simulink model "MotorCtrl_FOC_Math"  (R2025b)
settings: Solver=FixedStepDiscrete  StartTime=0.0  StopTime=5  FixedStep=MC_Sim_BaseStep  RelTol=1e-3  EnableMultiTasking=on
values from neighbouring files (symbols this model uses):
  MC_ADC_BitNum = 0.0    [MotorControlDataDictionary_Math.sldd]
  MC_ADC_Offset = 0.0    [MotorControlDataDictionary_Math.sldd]
  MC_ADC_VRef = 1.0    [MotorControlDataDictionary_Math.sldd]
  MC_CSA_Gain = 1.0    [MotorControlDataDictionary_Math.sldd]
  MC_MOS_DeadTime = 1.3E-6    [MotorControlDataDictionary_Math.sldd]
  MC_Motor_Mechinal_Damp = 1.0E-5    [MotorControlDataDictionary_Math.sldd]
  MC_Motor_Mechinal_Fric = 0.0    [MotorControlDataDictionary_Math.sldd]
  MC_Motor_Mechinal_Inertia = 0.0103    [MotorControlDataDictionary_Math.sldd]
  MC_Motor_Phi = 0.0059190254913385806    [MotorControlDataDictionary_Math.sldd]
  MC_Motor_Rotor_Pn = 4.0    [MotorControlDataDictionary_Math.sldd]
  MC_Motor_Stator_Ld = 5.6345E-5    [MotorControlDataDictionary_Math.sldd]
  MC_Motor_Stator_Lq = 5.6345E-5    [MotorControlDataDictionary_Math.sldd]
  MC_Motor_Stator_Rs = 0.0286    [MotorControlDataDictionary_Math.sldd]
  MC_Param_CurrentPI_Ki = 0.0089705790612839825    [MotorControlDataDictionary_Math.sldd]
  MC_Param_CurrentPI_Kp = 0.283220860906427    [MotorControlDataDictionary_Math.sldd]
  MC_Param_CurrentPI_UdInteMax = 7.794228634059948    [MotorControlDataDictionary_Math.sldd]
  MC_Param_CurrentPI_UdInteMin = -7.794228634059948    [MotorControlDataDictionary_Math.sldd]
  MC_Param_CurrentPI_UdMax = 7.794228634059948    [MotorControlDataDictionary_Math.sldd]
  MC_Param_CurrentPI_UdMin = -7.794228634059948    [MotorControlDataDictionary_Math.sldd]
  MC_Param_CurrentPI_UqInteMax = 7.794228634059948    [MotorControlDataDictionary_Math.sldd]
  MC_Param_CurrentPI_UqInteMin = -7.794228634059948    [MotorControlDataDictionary_Math.sldd]
  MC_Param_CurrentPI_UqMax = 7.794228634059948    [MotorControlDataDictionary_Math.sldd]
  MC_Param_CurrentPI_UqMin = -7.794228634059948    [MotorControlDataDictionary_Math.sldd]
  MC_Param_Flux_Gamma = 750000.0    [MotorControlDataDictionary_Math.sldd]
  MC_Param_Flux_Lalpha = 5.6345E-5    [MotorControlDataDictionary_Math.sldd]
  MC_Param_Flux_Lbeta = 5.6345E-5    [MotorControlDataDictionary_Math.sldd]
  MC_Param_Flux_Ralpha = 0.0286    [MotorControlDataDictionary_Math.sldd]
  MC_Param_Flux_Rbeta = 0.0286    [MotorControlDataDictionary_Math.sldd]
  MC_Param_Luen_BEMFalpha = -17747.803709290976    [MotorControlDataDictionary_Math.sldd]
  MC_Param_Luen_BEMFbeta = -17747.803709290976    [MotorControlDataDictionary_Math.sldd]
  MC_Param_Luen_BEMFErr = 10.0    [MotorControlDataDictionary_Math.sldd]
  MC_Param_Luen_Currentalpha = -507.58718608572195    [MotorControlDataDictionary_Math.sldd]
  MC_Param_Luen_Currentbeta = -507.58718608572195    [MotorControlDataDictionary_Math.sldd]
  MC_Param_Luen_CurrentErr = 400.0    [MotorControlDataDictionary_Math.sldd]
  MC_Param_Luen_PLL_Ki = 0.24634532585119037    [MotorControlDataDictionary_Math.sldd]
  MC_Param_Luen_PLL_Kp = 125.66370614359172    [MotorControlDataDictionary_Math.sldd]
  MC_Param_Luen_Voltagealpha = 17747.803709290976    [MotorControlDataDictionary_Math.sldd]
  MC_Param_Luen_Voltagebeta = 17747.803709290976    [MotorControlDataDictionary_Math.sldd]
  MC_Param_PhasetoReal = 500.0    [MotorControlDataDictionary_Math.sldd]
  MC_Param_SMO_CoffA = 0.968326559588251    [MotorControlDataDictionary_Math.sldd]
  MC_Param_SMO_CoffB = 1.1074629514597569    [MotorControlDataDictionary_Math.sldd]
  MC_Param_SpeedCtrl_IdMax = 60.0    [MotorControlDataDictionary_Math.sldd]
  MC_Param_SpeedCtrl_IdMin = -60.0    [MotorControlDataDictionary_Math.sldd]
  MC_Param_SpeedCtrl_IqMax = 60.0    [MotorControlDataDictionary_Math.sldd]
  MC_Param_SpeedCtrl_IqMin = -60.0    [MotorControlDataDictionary_Math.sldd]
  MC_Param_SpeedPI_Ki = 0.57157085739428382    [MotorControlDataDictionary_Math.sldd]
  MC_Param_SpeedPI_Kp = 9.1114109857344836    [MotorControlDataDictionary_Math.sldd]
  MC_Param_SpeedtoTheta = 6.24E-5    [MotorControlDataDictionary_Math.sldd]
  MC_Param_SVPWM_DutyMax = 0.98    [MotorControlDataDictionary_Math.sldd]
  MC_Param_SVPWM_DutyMin = 0.02    [MotorControlDataDictionary_Math.sldd]
  MC_Param_SVPWM_SampleOffset1 = 0.02    [MotorControlDataDictionary_Math.sldd]
  MC_Param_SVPWM_SampleOffset2 = 0.015    [MotorControlDataDictionary_Math.sldd]
  MC_Param_SVPWM_SampleValid = 0.0096153846153846159    [MotorControlDataDictionary_Math.sldd]
  MC_Param_Zero = 0.0    [MotorControlDataDictionary_Math.sldd]
  MC_Sample_CurrentNoise = 1.0E-15    [MotorControlDataDictionary_Math.sldd]
  MC_Sample_Rs = 0.002    [MotorControlDataDictionary_Math.sldd]
  MC_Sample_VbusNoise = 1.0E-15    [MotorControlDataDictionary_Math.sldd]
  MC_Sim_BaseStep = 2.08E-8    [MotorControlDataDictionary_Math.sldd]
  MC_Sim_HFTStep = 6.24E-5    [MotorControlDataDictionary_Math.sldd]
  MC_Sim_MFTStep = 0.0019968    [MotorControlDataDictionary_Math.sldd]
libraries: simulink x28, nesl_utility x19, fl_lib x14, ee_lib x13, autolibpmsminterior x2, autolibinverter x1
(part 2 of 8)

== system MotorCtrl_FOC_Math/Tracking-Differentiator ==
  Ref_In : Inport
  Add : Sum
  Add1 : Sum
  Delay One Step : Delay  DelayLength=1  InitialCondition=MC_Param_Zero
  Delay One Step1 : Delay  DelayLength=1  InitialCondition=MC_Param_Zero
  Gain : Gain  Gain=MC_Sim_MFTStep  ParamDataTypeStr=single  OutDataTypeStr=single  RndMeth=Simplest
  Gain1 : Gain  Gain=MC_Sim_MFTStep  OutDataTypeStr=single  RndMeth=Simplest
  Signal Copy : SignalConversion  OverrideOpt=off
  fastFunc1_TD : Subsystem  Commented=on
  fastFunc2_TD : Subsystem
  SpeedTarget_TD : Outport
  wires:
  Ref_In/1 -> fastFunc2_TD/1(Ref_In), fastFunc1_TD/1(Ref_In)
  fastFunc2_TD/1(Ref_TD) -> Gain/1  "u"
  Add/1 -> Gain1/1, Delay One Step/1  "x2"
  Delay One Step/1 -> Add/2, [x2_delay]
  Gain/1 -> Add/1  "T*u"
  Gain1/1 -> Add1/1  "T*x2"
  Add1/1 -> Signal Copy/1, Delay One Step1/1  "x1"
  Delay One Step1/1 -> Add1/2, [x1_delay]
  Signal Copy/1 -> SpeedTarget_TD/1  "SpeedTarget_TD"
  [x1_delay] -> fastFunc2_TD/2(X1), fastFunc1_TD/2(X1)
  [x2_delay] -> fastFunc2_TD/3(X2), fastFunc1_TD/3(X2)

== system MotorCtrl_FOC_Math/HFTask/LuenbergerObservor ==
  Valpha : Inport
  Vbeta : Inport  Port=2
  Ialpha : Inport  Port=3
  Ibeta : Inport  Port=4
  We : Inport  Port=5
  Delay One Step : Delay  DelayLength=1  InitialCondition=single(0)
  Terminator : Terminator
  getE : Subsystem
  getSpeedandTheta : Subsystem
  Speed : Outport
  Theta : Outport  Port=2
  wires:
  getSpeedandTheta/2(Theta) -> Theta/1
  getSpeedandTheta/1(Speed) -> Speed/1
  getE/2(Ebeta) -> getSpeedandTheta/2(Ebeta)
  getE/1(Ealpha) -> getSpeedandTheta/1(Ealpha)
  Ibeta/1 -> getE/4(Ibeta)
  Ialpha/1 -> getE/3(Ialpha)
  Vbeta/1 -> getE/2(Vbeta)
  Valpha/1 -> getE/1(Valpha)
  getSpeedandTheta/3(We) -> Delay One Step/1
  We/1 -> Terminator/1
  Delay One Step/1 -> getE/5(We)

== system MotorCtrl_FOC_Math/HFTask/axisTransform ==
  Ia : Inport
  Ib : Inport  Port=2
  SinTheta : Inport  Port=3
  CosTheta : Inport  Port=4
  Add1 : Sum
  Product{,1..3} (4 alike) : Product
  Signal Copy : SignalConversion  OverrideOpt=off
  Subtract : Sum  Inputs=-+
  a_plus_2b : Sum  Inputs=+++  RndMeth=Simplest  OutDataTypeStr=Inherit: Same as first input
  one_by_sqrt3 : Gain  Gain=1/sqrt(3)  RndMeth=Simplest  OutDataTypeStr=Inherit: Same as input
  Ialpha : Outport
  Ibeta : Outport  Port=2
  Id : Outport  Port=3
  Iq : Outport  Port=4
  wires:
  Product3/1 -> Subtract/2
  Product2/1 -> Subtract/1
  Add1/1 -> Id/1  "Id"
  Subtract/1 -> Iq/1  "Iq"
  Product/1 -> Add1/1
  Product1/1 -> Add1/2
  CosTheta/1 -> Product3/2, Product/2
  SinTheta/1 -> Product2/2, Product1/2
  a_plus_2b/1 -> one_by_sqrt3/1
  one_by_sqrt3/1 -> Ibeta/1, Product3/1, Product1/1  "Ibeta"
  Signal Copy/1 -> Ialpha/1, Product2/1, Product/1  "Ialpha"
  Ia/1 -> a_plus_2b/1, Signal Copy/1
  Ib/1 -> a_plus_2b/3, a_plus_2b/2

== system MotorCtrl_FOC_Math/HFTask/currentADRC ==
  note: ADRC开发日志:
      | 20251229：
      | 感觉观测器参数存在问题，观测值瞬间会和参考值相等，导致PI控制器调节电流增速较慢
      | 2026.01.05
      | 1、LESO中的两个fal函数出现周期性震荡
      | 2、NLSEF中的电压输出值只有1.xV，电机转速无法提升
      | 2026.01.07
      | 1、减小NLSEF的参数，可以实现系统的收敛，且效果与PI控制器类似
  IdRef : Inport
  IqRef : Inport  Port=2
  Id : Inport  Port=3
  Iq : Inport  Port=4
  Ud : Inport  Port=5
  Uq : Inport  Port=6
  IntregralResetFlag : Inport  Port=7
  Wm : Inport  Port=8
  Delay One Step : Delay  InitialCondition=single(0)
  Delay One Step1 : Delay  InitialCondition=single(0)
  LESO : Subsystem  VariantControl=ESO
  NLSEF : Subsystem  VariantControl=NLSEF
  Terminator : Terminator
  UdRef : Outport
  UqRef : Outport  Port=2
  wires:
  NLSEF/1(Ud_ADRC) -> UdRef/1  "UdRef"
  NLSEF/2(Uq_ADRC) -> UqRef/1  "UqRef"
  IdRef/1 -> NLSEF/1(Id_Ref)
  Id/1 -> LESO/1(Id)
  IqRef/1 -> NLSEF/2(Iq_Ref)
  Iq/1 -> LESO/3(Iq)
  IntregralResetFlag/1 -> Terminator/1
  Delay One Step/1 -> LESO/2(Ud)
  Delay One Step1/1 -> LESO/4(Uq)
  LESO/2(Iq_ESO) -> NLSEF/4(Iq_ESO)
  LESO/1(Id_ESO) -> NLSEF/3(Id_ESO)
  LESO/3(Id_Dis) -> NLSEF/5(Id_ESO_Dis)
  LESO/4(Iq_Dis) -> NLSEF/6(Iq_ESO_Dis)
  Ud/1 -> Delay One Step/1
  Uq/1 -> Delay One Step1/1

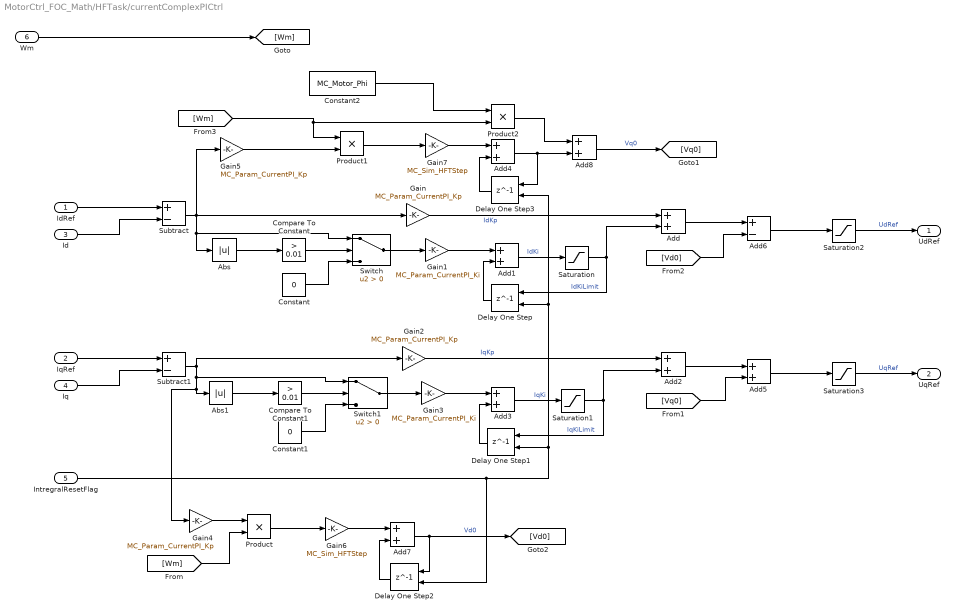
== system MotorCtrl_FOC_Math/HFTask/currentComplexPICtrl ==
  IdRef : Inport
  IqRef : Inport  Port=2
  Id : Inport  Port=3
  Iq : Inport  Port=4
  IntregralResetFlag : Inport  Port=5
  Wm : Inport  Port=6
  Abs : Abs  SaturateOnIntegerOverflow=off
  Abs1 : Abs  SaturateOnIntegerOverflow=off
  Add{,2,5,8} (4 alike) : Sum
  Add{1,3..4,7} (4 alike) : Sum  OutDataTypeStr=single
  Add6 : Sum  Inputs=+-
  Compare To Constant : simulink/Logic and Bit Operations/Compare To Constant  relop=>  const=0.01  OutDataTypeStr=boolean
  Compare To Constant1 : simulink/Logic and Bit Operations/Compare To Constant  relop=>  const=0.01  OutDataTypeStr=boolean
  Constant : Constant  Value=0  OutDataTypeStr=single
  Constant1 : Constant  Value=0  OutDataTypeStr=single
  Constant2 : Constant  Value=MC_Motor_Phi  OutDataTypeStr=single
  Delay One Step{,1..3} (4 alike) : Delay  DelayLength=1  ExternalReset=Level
      settings: InputPortMap=u0,r5
  Gain : Gain  Gain=MC_Param_CurrentPI_Kp  OutDataTypeStr=single
  Gain1 : Gain  Gain=MC_Param_CurrentPI_Ki  OutDataTypeStr=single
  Gain2 : Gain  Gain=MC_Param_CurrentPI_Kp  OutDataTypeStr=single
  Gain3 : Gain  Gain=MC_Param_CurrentPI_Ki  OutDataTypeStr=single
  Gain4 : Gain  Gain=MC_Param_CurrentPI_Kp
  Gain5 : Gain  Gain=MC_Param_CurrentPI_Kp
  Gain6 : Gain  Gain=MC_Sim_HFTStep  OutDataTypeStr=single
  Gain7 : Gain  Gain=MC_Sim_HFTStep  OutDataTypeStr=single
  Product : Product
  Product1 : Product
  Product2 : Product
  Saturation : Saturate  UpperLimit=MC_Param_CurrentPI_UdInteMax  LowerLimit=MC_Param_CurrentPI_UdInteMin
  Saturation1 : Saturate  UpperLimit=MC_Param_CurrentPI_UqInteMax  LowerLimit=MC_Param_CurrentPI_UqInteMin
  Saturation2 : Saturate  UpperLimit=MC_Param_CurrentPI_UdMax  LowerLimit=MC_Param_CurrentPI_UdMin
  Saturation3 : Saturate  UpperLimit=MC_Param_CurrentPI_UqMax  LowerLimit=MC_Param_CurrentPI_UqMin
  Subtract : Sum  Inputs=+-
  Subtract1 : Sum  Inputs=+-
  Switch : Switch  Criteria=u2 > Threshold  SaturateOnIntegerOverflow=off  InputSameDT=off
  Switch1 : Switch  Criteria=u2 > Threshold  SaturateOnIntegerOverflow=off  InputSameDT=off
  UdRef : Outport
  UqRef : Outport  Port=2
  wires:
  Wm/1 -> [Wm]
  Saturation3/1 -> UqRef/1  "UqRef"
  Saturation2/1 -> UdRef/1  "UdRef"
  [Vd0] -> Add6/2
  Add6/1 -> Saturation2/1
  Add/1 -> Add6/1
  [Vq0] -> Add5/2
  Add2/1 -> Add5/1
  [Wm] -> Product/2
  Id/1 -> Subtract/2
  Gain4/1 -> Product/1
  Switch1/1 -> Gain3/1
  Abs1/1 -> Compare To Constant1/1
  Compare To Constant1/1 -> Switch1/2
  Constant1/1 -> Switch1/3
  Constant/1 -> Switch/3
  Compare To Constant/1 -> Switch/2
  Switch/1 -> Gain1/1
  Add5/1 -> Saturation3/1
  IqRef/1 -> Subtract1/1
  Iq/1 -> Subtract1/2
  Subtract1/1 -> Gain2/1, Gain4/1, Abs1/1, Switch1/1
  Gain2/1 -> Add2/1  "IqKp"
  Gain3/1 -> Add3/1
  Delay One Step1/1 -> Add3/2
  Add3/1 -> Saturation1/1  "IqKi"
  Saturation1/1 -> Add2/2, Delay One Step1/1  "IqKiLimit"
  Saturation/1 -> Delay One Step/1, Add/2  "IdKiLimit"
  Add1/1 -> Saturation/1  "IdKi"
  Delay One Step/1 -> Add1/2
  Gain1/1 -> Add1/1
  Abs/1 -> Compare To Constant/1
  Gain/1 -> Add/1  "IdKp"
  Subtract/1 -> Gain5/1, Abs/1, Switch/1, Gain/1
  IdRef/1 -> Subtract/1
  Gain6/1 -> Add7/1
  Product/1 -> Gain6/1
  Delay One Step2/1 -> Add7/2
  Add7/1 -> [Vd0], Delay One Step2/1  "Vd0"
  Add4/1 -> Delay One Step3/1, Add8/2
  Delay One Step3/1 -> Add4/2
  Gain7/1 -> Add4/1
  IntregralResetFlag/1 -> Delay One Step2/2, Delay One Step1/2, Delay One Step3/2, Delay One Step/2
  Product1/1 -> Gain7/1
  Constant2/1 -> Product2/1
  Gain5/1 -> Product1/2
  Add8/1 -> [Vq0]  "Vq0"
  Product2/1 -> Add8/1
  [Wm] -> Product1/1, Product2/2

== system MotorCtrl_FOC_Math/HFTask/currentDBC ==
  note: 无差拍电流控制器（延时1拍）
  IdRef : Inport
  IqRef : Inport  Port=2
  Id : Inport  Port=3
  Iq : Inport  Port=4
  Wm : Inport  Port=5
  Add5 : Sum  Inputs=++-
  Add6 : Sum  Inputs=+++
  Add7 : Sum
  Constant1 : Constant  Value=MC_Motor_Phi  OutDataTypeStr=single
  Gain10 : Gain  Gain=MC_Motor_Stator_Lq
  Gain11 : Gain  Gain=MC_Motor_Stator_Lq/MC_Sim_HFTStep
  Gain12 : Gain  Gain=MC_Motor_Stator_Rs-(MC_Motor_Stator_Lq/MC_Sim_HFTStep)
  Gain13 : Gain  Gain=MC_Motor_Stator_Ld
  Gain8 : Gain  Gain=MC_Motor_Stator_Ld/MC_Sim_HFTStep
  Gain9 : Gain  Gain=MC_Motor_Stator_Rs-(MC_Motor_Stator_Ld/MC_Sim_HFTStep)
  Product2 : Product
  Product3 : Product
  Saturation : Saturate  UpperLimit=MC_Param_CurrentPI_UdMax  LowerLimit=MC_Param_CurrentPI_UdMin
  Saturation1 : Saturate  UpperLimit=MC_Param_CurrentPI_UqMax  LowerLimit=MC_Param_CurrentPI_UqMin
  UdRef : Outport
  UqRef : Outport  Port=2
  wires:
  Wm/1 -> [Wm]
  Iq/1 -> [Iq]
  Id/1 -> [Id]
  IqRef/1 -> [IqRef]
  IdRef/1 -> [IdRef]
  [IdRef] -> Gain8/1
  Gain8/1 -> Add5/1  "IdRef_Vd"
  [Id] -> Gain9/1
  Gain9/1 -> Add5/2  "Id_Vd"
  [Iq] -> Gain10/1
  Gain10/1 -> Product2/2
  [Wm] -> Product2/1
  [IqRef] -> Gain11/1
  Gain11/1 -> Add6/1  "IqRef_Vq"
  Gain12/1 -> Add6/2  "Iq_Vq"
  [Iq] -> Gain12/1
  [Wm] -> Product3/1
  Add7/1 -> Product3/2
  Constant1/1 -> Add7/2
  Gain13/1 -> Add7/1
  [Id] -> Gain13/1
  Saturation/1 -> UdRef/1  "UdRef_DBC"
  Saturation1/1 -> UqRef/1  "UqRef_DBC"
  Add5/1 -> Saturation/1
  Product2/1 -> Add5/3  "Iq_Vd"
  Add6/1 -> Saturation1/1
  Product3/1 -> Add6/3  "Id_Vq"

== system MotorCtrl_FOC_Math/HFTask/currentPIControl ==
  IdRef : Inport
  IqRef : Inport  Port=2
  Id : Inport  Port=3
  Iq : Inport  Port=4
  IntregralResetFlag : Inport  Port=5
  Wm : Inport  Port=6
  Abs : Abs  SaturateOnIntegerOverflow=off
  Abs1 : Abs  SaturateOnIntegerOverflow=off
  Add{,2,4..5} (4 alike) : Sum
  Add1 : Sum  OutDataTypeStr=single
  Add3 : Sum  OutDataTypeStr=single
  Add6 : Sum  Inputs=+-
  Compare To Constant : simulink/Logic and Bit Operations/Compare To Constant  relop=>  const=0.01  OutDataTypeStr=boolean
  Compare To Constant1 : simulink/Logic and Bit Operations/Compare To Constant  relop=>  const=0.01  OutDataTypeStr=boolean
  Constant : Constant  Value=0  OutDataTypeStr=single
  Constant1 : Constant  Value=0  OutDataTypeStr=single
  Constant2 : Constant  Value=MC_Motor_Phi  OutDataTypeStr=single
  Delay One Step : Delay  DelayLength=1  ExternalReset=Level
      settings: InputPortMap=u0,r5
  Delay One Step1 : Delay  DelayLength=1  ExternalReset=Level
      settings: InputPortMap=u0,r5
  Gain : Gain  Gain=MC_Param_CurrentPI_Kp  OutDataTypeStr=single
  Gain1 : Gain  Gain=MC_Param_CurrentPI_Ki  OutDataTypeStr=single
  Gain2 : Gain  Gain=MC_Param_CurrentPI_Kp  OutDataTypeStr=single
  Gain3 : Gain  Gain=MC_Param_CurrentPI_Ki  OutDataTypeStr=single
  Gain4 : Gain  Gain=MC_Motor_Stator_Lq
  Gain5 : Gain  Gain=MC_Motor_Stator_Ld
  Product : Product
  Product1 : Product
  Saturation : Saturate  UpperLimit=MC_Param_CurrentPI_UdInteMax  LowerLimit=MC_Param_CurrentPI_UdInteMin
  Saturation1 : Saturate  UpperLimit=MC_Param_CurrentPI_UqInteMax  LowerLimit=MC_Param_CurrentPI_UqInteMin
  Saturation2 : Saturate  UpperLimit=MC_Param_CurrentPI_UdMax  LowerLimit=MC_Param_CurrentPI_UdMin
  Saturation3 : Saturate  UpperLimit=MC_Param_CurrentPI_UqMax  LowerLimit=MC_Param_CurrentPI_UqMin
  Subtract : Sum  Inputs=+-
  Subtract1 : Sum  Inputs=+-
  Switch : Switch  Criteria=u2 > Threshold  SaturateOnIntegerOverflow=off  InputSameDT=off
  Switch1 : Switch  Criteria=u2 > Threshold  SaturateOnIntegerOverflow=off  InputSameDT=off
  UdRef : Outport
  UqRef : Outport  Port=2
  wires:
  IdRef/1 -> Subtract/1
  Subtract/1 -> Gain/1, Switch/1, Abs/1
  Gain/1 -> Add/1  "IdKp"
  Abs/1 -> Compare To Constant/1
  Gain1/1 -> Add1/1
  Delay One Step/1 -> Add1/2
  Add1/1 -> Saturation/1  "IdKi"
  Saturation/1 -> Add/2, Delay One Step/1  "IdKiLimit"
  Saturation1/1 -> Delay One Step1/1, Add2/2  "IqKiLimit"
  Add3/1 -> Saturation1/1  "IqKi"
  Delay One Step1/1 -> Add3/2
  Gain3/1 -> Add3/1
  Gain2/1 -> Add2/1  "IqKp"
  Subtract1/1 -> Switch1/1, Abs1/1, Gain2/1
  Iq/1 -> Gain4/1, Subtract1/2
  IqRef/1 -> Subtract1/1
  IntregralResetFlag/1 -> Delay One Step/2, Delay One Step1/2
  Add5/1 -> Saturation3/1
  Switch/1 -> Gain1/1
  Compare To Constant/1 -> Switch/2
  Constant/1 -> Switch/3
  Constant1/1 -> Switch1/3
  Compare To Constant1/1 -> Switch1/2
  Abs1/1 -> Compare To Constant1/1
  Switch1/1 -> Gain3/1
  Gain4/1 -> Product/1
  Id/1 -> Gain5/1, Subtract/2
  [Wm] -> Product/2
  Gain5/1 -> Add4/1
  Add4/1 -> Product1/2
  Constant2/1 -> Add4/2
  Product1/1 -> [Vq0]
  Product/1 -> [Vd0]
  Add2/1 -> Add5/1
  [Vq0] -> Add5/2
  Add/1 -> Add6/1
  Add6/1 -> Saturation2/1
  [Vd0] -> Add6/2
  Saturation2/1 -> UdRef/1  "UdRef"
  Saturation3/1 -> UqRef/1  "UqRef"
  [Wm] -> Product1/1
  Wm/1 -> [Wm]

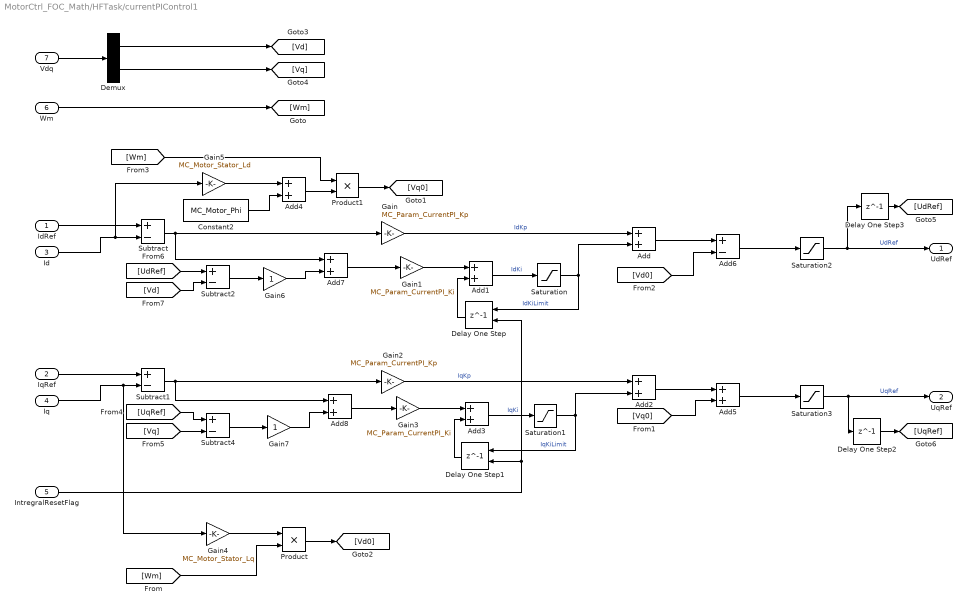
== system MotorCtrl_FOC_Math/HFTask/currentPIControl1 ==
  IdRef : Inport
  IqRef : Inport  Port=2
  Id : Inport  Port=3
  Iq : Inport  Port=4
  IntregralResetFlag : Inport  Port=5
  Wm : Inport  Port=6
  Vdq : Inport  Port=7
  Add{,2,4..5,7..8} (6 alike) : Sum
  Add1 : Sum  OutDataTypeStr=single
  Add3 : Sum  OutDataTypeStr=single
  Add6 : Sum  Inputs=+-
  Constant2 : Constant  Value=MC_Motor_Phi  OutDataTypeStr=single
  Delay One Step : Delay  DelayLength=1  ExternalReset=Level
      settings: InputPortMap=u0,r5
  Delay One Step1 : Delay  DelayLength=1  ExternalReset=Level
      settings: InputPortMap=u0,r5
  Delay One Step2 : Delay  DelayLength=1  InitialCondition=single(0)
  Delay One Step3 : Delay  DelayLength=1  InitialCondition=single(0)
  Demux : Demux  Outputs=2
  Gain : Gain  Gain=MC_Param_CurrentPI_Kp  OutDataTypeStr=single
  Gain1 : Gain  Gain=MC_Param_CurrentPI_Ki  OutDataTypeStr=single
  Gain2 : Gain  Gain=MC_Param_CurrentPI_Kp  OutDataTypeStr=single
  Gain3 : Gain  Gain=MC_Param_CurrentPI_Ki  OutDataTypeStr=single
  Gain4 : Gain  Gain=MC_Motor_Stator_Lq
  Gain5 : Gain  Gain=MC_Motor_Stator_Ld
  Gain6 : Gain
  Gain7 : Gain
  Product : Product
  Product1 : Product
  Saturation : Saturate  UpperLimit=MC_Param_CurrentPI_UdInteMax  LowerLimit=MC_Param_CurrentPI_UdInteMin
  Saturation1 : Saturate  UpperLimit=MC_Param_CurrentPI_UqInteMax  LowerLimit=MC_Param_CurrentPI_UqInteMin
  Saturation2 : Saturate  UpperLimit=MC_Param_CurrentPI_UdMax  LowerLimit=MC_Param_CurrentPI_UdMin
  Saturation3 : Saturate  UpperLimit=MC_Param_CurrentPI_UqMax  LowerLimit=MC_Param_CurrentPI_UqMin
  Subtract{,1..2,4} (4 alike) : Sum  Inputs=+-
  UdRef : Outport
  UqRef : Outport  Port=2
  wires:
  Wm/1 -> [Wm]
  [Wm] -> Product1/1
  Saturation3/1 -> Delay One Step2/1, UqRef/1  "UqRef"
  Saturation2/1 -> Delay One Step3/1, UdRef/1  "UdRef"
  [Vd0] -> Add6/2
  Add6/1 -> Saturation2/1
  Add/1 -> Add6/1
  [Vq0] -> Add5/2
  Add2/1 -> Add5/1
  Product/1 -> [Vd0]
  Product1/1 -> [Vq0]
  Constant2/1 -> Add4/2
  Add4/1 -> Product1/2
  Gain5/1 -> Add4/1
  [Wm] -> Product/2
  Id/1 -> Subtract/2, Gain5/1
  Gain4/1 -> Product/1
  Add8/1 -> Gain3/1
  Add5/1 -> Saturation3/1
  IntregralResetFlag/1 -> Delay One Step1/2, Delay One Step/2
  IqRef/1 -> Subtract1/1
  Iq/1 -> Subtract1/2, Gain4/1
  Subtract1/1 -> Add8/1, Gain2/1
  Gain2/1 -> Add2/1  "IqKp"
  Gain3/1 -> Add3/1
  Delay One Step1/1 -> Add3/2
  Add3/1 -> Saturation1/1  "IqKi"
  Saturation1/1 -> Add2/2, Delay One Step1/1  "IqKiLimit"
  Saturation/1 -> Delay One Step/1, Add/2  "IdKiLimit"
  Add1/1 -> Saturation/1  "IdKi"
  Delay One Step/1 -> Add1/2
  Gain1/1 -> Add1/1
  Gain/1 -> Add/1  "IdKp"
  Subtract/1 -> Add7/1, Gain/1
  IdRef/1 -> Subtract/1
  Vdq/1 -> Demux/1
  Demux/1 -> [Vd]
  Demux/2 -> [Vq]
  Add7/1 -> Gain1/1
  [Vq] -> Subtract4/2
  [UqRef] -> Subtract4/1
  Subtract2/1 -> Gain6/1
  Gain6/1 -> Add7/2
  Subtract4/1 -> Gain7/1
  Gain7/1 -> Add8/2
  [UdRef] -> Subtract2/1
  [Vd] -> Subtract2/2
  Delay One Step2/1 -> [UqRef]
  Delay One Step3/1 -> [UdRef]

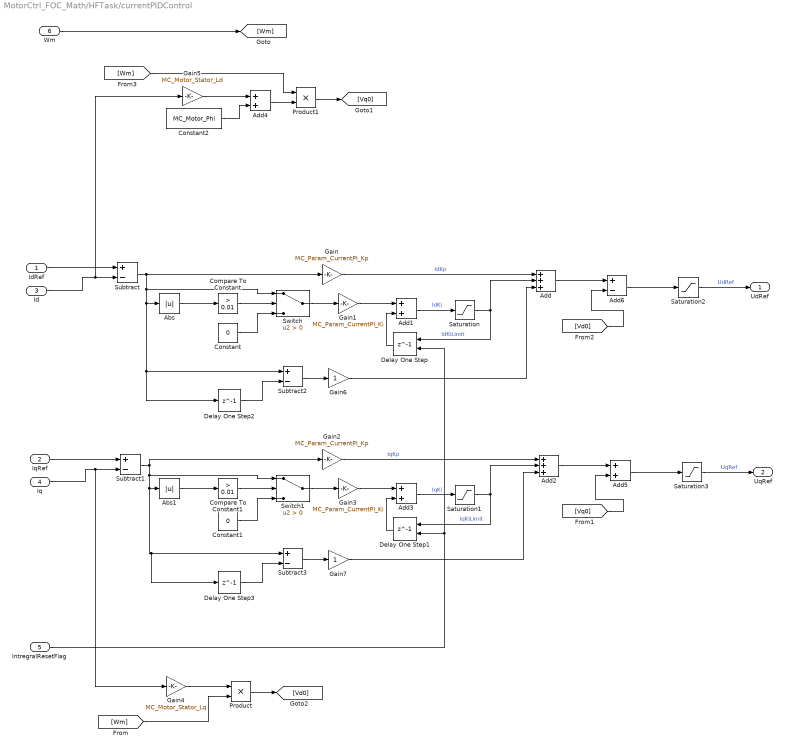
== system MotorCtrl_FOC_Math/HFTask/currentPIDControl ==
  IdRef : Inport
  IqRef : Inport  Port=2
  Id : Inport  Port=3
  Iq : Inport  Port=4
  IntregralResetFlag : Inport  Port=5
  Wm : Inport  Port=6
  Abs : Abs  SaturateOnIntegerOverflow=off
  Abs1 : Abs  SaturateOnIntegerOverflow=off
  Add : Sum  Inputs=+++
  Add1 : Sum  OutDataTypeStr=single
  Add2 : Sum  Inputs=+++
  Add3 : Sum  OutDataTypeStr=single
  Add4 : Sum
  Add5 : Sum
  Add6 : Sum  Inputs=+-
  Compare To Constant : simulink/Logic and Bit Operations/Compare To Constant  relop=>  const=0.01  OutDataTypeStr=boolean
  Compare To Constant1 : simulink/Logic and Bit Operations/Compare To Constant  relop=>  const=0.01  OutDataTypeStr=boolean
  Constant : Constant  Value=0  OutDataTypeStr=single
  Constant1 : Constant  Value=0  OutDataTypeStr=single
  Constant2 : Constant  Value=MC_Motor_Phi  OutDataTypeStr=single
  Delay One Step : Delay  DelayLength=1  ExternalReset=Level
      settings: InputPortMap=u0,r5
  Delay One Step1 : Delay  DelayLength=1  ExternalReset=Level
      settings: InputPortMap=u0,r5
  Delay One Step2 : Delay  DelayLength=1  InitialCondition=single(0)
  Delay One Step3 : Delay  DelayLength=1  InitialCondition=single(0)
  Gain : Gain  Gain=MC_Param_CurrentPI_Kp  OutDataTypeStr=single
  Gain1 : Gain  Gain=MC_Param_CurrentPI_Ki  OutDataTypeStr=single
  Gain2 : Gain  Gain=MC_Param_CurrentPI_Kp  OutDataTypeStr=single
  Gain3 : Gain  Gain=MC_Param_CurrentPI_Ki  OutDataTypeStr=single
  Gain4 : Gain  Gain=MC_Motor_Stator_Lq
  Gain5 : Gain  Gain=MC_Motor_Stator_Ld
  Gain6 : Gain
  Gain7 : Gain
  Product : Product
  Product1 : Product
  Saturation : Saturate  UpperLimit=MC_Param_CurrentPI_UdInteMax  LowerLimit=MC_Param_CurrentPI_UdInteMin
  Saturation1 : Saturate  UpperLimit=MC_Param_CurrentPI_UqInteMax  LowerLimit=MC_Param_CurrentPI_UqInteMin
  Saturation2 : Saturate  UpperLimit=MC_Param_CurrentPI_UdMax  LowerLimit=MC_Param_CurrentPI_UdMin
  Saturation3 : Saturate  UpperLimit=MC_Param_CurrentPI_UqMax  LowerLimit=MC_Param_CurrentPI_UqMin
  Subtract{,1..3} (4 alike) : Sum  Inputs=+-
  Switch : Switch  Criteria=u2 > Threshold  SaturateOnIntegerOverflow=off  InputSameDT=off
  Switch1 : Switch  Criteria=u2 > Threshold  SaturateOnIntegerOverflow=off  InputSameDT=off
  UdRef : Outport
  UqRef : Outport  Port=2
  wires:
  IdRef/1 -> Subtract/1
  Subtract/1 -> Gain/1, Switch/1, Subtract2/1, Delay One Step2/1, Abs/1
  Gain/1 -> Add/1  "IdKp"
  Abs/1 -> Compare To Constant/1
  Gain1/1 -> Add1/1
  Delay One Step/1 -> Add1/2
  Add1/1 -> Saturation/1  "IdKi"
  Saturation/1 -> Add/2, Delay One Step/1  "IdKiLimit"
  Saturation1/1 -> Delay One Step1/1, Add2/2  "IqKiLimit"
  Add3/1 -> Saturation1/1  "IqKi"
  Delay One Step1/1 -> Add3/2
  Gain3/1 -> Add3/1
  Gain2/1 -> Add2/1  "IqKp"
  Iq/1 -> Subtract1/2, Gain4/1
  IqRef/1 -> Subtract1/1
  IntregralResetFlag/1 -> Delay One Step/2, Delay One Step1/2
  Add5/1 -> Saturation3/1
  Switch/1 -> Gain1/1
  Compare To Constant/1 -> Switch/2
  Constant/1 -> Switch/3
  Constant1/1 -> Switch1/3
  Compare To Constant1/1 -> Switch1/2
  Abs1/1 -> Compare To Constant1/1
  Switch1/1 -> Gain3/1
  Gain4/1 -> Product/1
  Id/1 -> Gain5/1, Subtract/2
  [Wm] -> Product/2
  Gain5/1 -> Add4/1
  Add4/1 -> Product1/2
  Constant2/1 -> Add4/2
  Product1/1 -> [Vq0]
  Product/1 -> [Vd0]
  Add2/1 -> Add5/1
  [Vq0] -> Add5/2
  Add/1 -> Add6/1
  Add6/1 -> Saturation2/1
  [Vd0] -> Add6/2
  Saturation2/1 -> UdRef/1  "UdRef"
  Saturation3/1 -> UqRef/1  "UqRef"
  [Wm] -> Product1/1
  Wm/1 -> [Wm]
  Delay One Step2/1 -> Subtract2/2
  Subtract2/1 -> Gain6/1
  Gain6/1 -> Add/3
  Gain7/1 -> Add2/3
  Subtract3/1 -> Gain7/1
  Delay One Step3/1 -> Subtract3/2
  Subtract1/1 -> Switch1/1, Delay One Step3/1, Subtract3/1, Abs1/1, Gain2/1

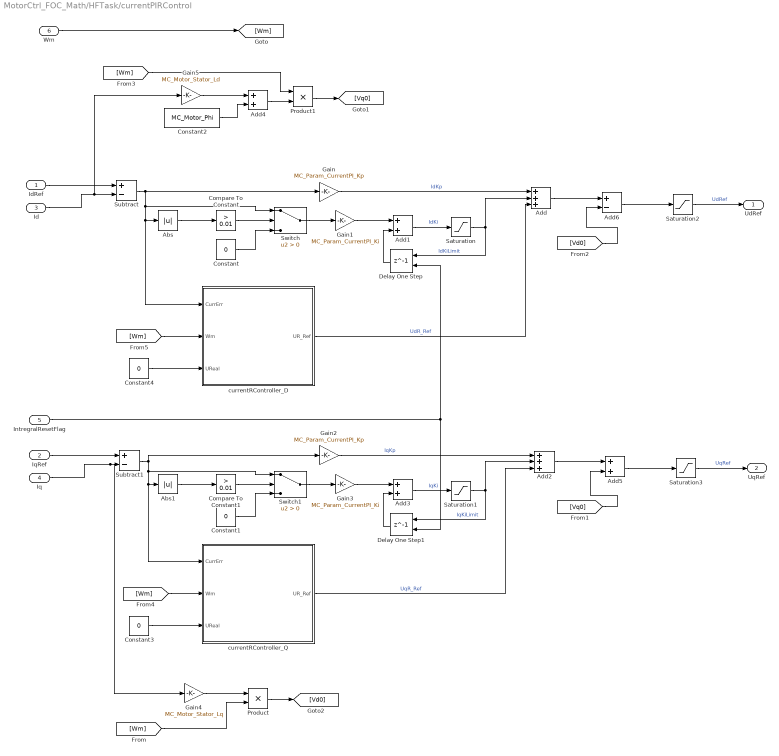
== system MotorCtrl_FOC_Math/HFTask/currentPIRControl ==
  IdRef : Inport
  IqRef : Inport  Port=2
  Id : Inport  Port=3
  Iq : Inport  Port=4
  IntregralResetFlag : Inport  Port=5
  Wm : Inport  Port=6
  Abs : Abs  SaturateOnIntegerOverflow=off
  Abs1 : Abs  SaturateOnIntegerOverflow=off
  Add : Sum  Inputs=+++
  Add1 : Sum  OutDataTypeStr=single
  Add2 : Sum  Inputs=+++
  Add3 : Sum  OutDataTypeStr=single
  Add4 : Sum
  Add5 : Sum
  Add6 : Sum  Inputs=+-
  Compare To Constant : simulink/Logic and Bit Operations/Compare To Constant  relop=>  const=0.01  OutDataTypeStr=boolean
  Compare To Constant1 : simulink/Logic and Bit Operations/Compare To Constant  relop=>  const=0.01  OutDataTypeStr=boolean
  Constant{,1,3..4} (4 alike) : Constant  Value=0  OutDataTypeStr=single
  Constant2 : Constant  Value=MC_Motor_Phi  OutDataTypeStr=single
  Delay One Step : Delay  DelayLength=1  ExternalReset=Level
      settings: InputPortMap=u0,r5
  Delay One Step1 : Delay  DelayLength=1  ExternalReset=Level
      settings: InputPortMap=u0,r5
  Gain : Gain  Gain=MC_Param_CurrentPI_Kp  OutDataTypeStr=single
  Gain1 : Gain  Gain=MC_Param_CurrentPI_Ki  OutDataTypeStr=single
  Gain2 : Gain  Gain=MC_Param_CurrentPI_Kp  OutDataTypeStr=single
  Gain3 : Gain  Gain=MC_Param_CurrentPI_Ki  OutDataTypeStr=single
  Gain4 : Gain  Gain=MC_Motor_Stator_Lq
  Gain5 : Gain  Gain=MC_Motor_Stator_Ld
  Product : Product
  Product1 : Product
  Saturation : Saturate  UpperLimit=MC_Param_CurrentPI_UdInteMax  LowerLimit=MC_Param_CurrentPI_UdInteMin
  Saturation1 : Saturate  UpperLimit=MC_Param_CurrentPI_UqInteMax  LowerLimit=MC_Param_CurrentPI_UqInteMin
  Saturation2 : Saturate  UpperLimit=MC_Param_CurrentPI_UdMax  LowerLimit=MC_Param_CurrentPI_UdMin
  Saturation3 : Saturate  UpperLimit=MC_Param_CurrentPI_UqMax  LowerLimit=MC_Param_CurrentPI_UqMin
  Subtract : Sum  Inputs=+-
  Subtract1 : Sum  Inputs=+-
  Switch : Switch  Criteria=u2 > Threshold  SaturateOnIntegerOverflow=off  InputSameDT=off
  Switch1 : Switch  Criteria=u2 > Threshold  SaturateOnIntegerOverflow=off  InputSameDT=off
  currentRController_D : Subsystem
  currentRController_Q : Subsystem
  UdRef : Outport
  UqRef : Outport  Port=2
  wires:
  Subtract1/1 -> Gain2/1, currentRController_Q/1(CurrErr), Abs1/1, Switch1/1
  Wm/1 -> [Wm]
  [Wm] -> Product1/1
  Saturation3/1 -> UqRef/1  "UqRef"
  Saturation2/1 -> UdRef/1  "UdRef"
  [Vd0] -> Add6/2
  Add6/1 -> Saturation2/1
  Add/1 -> Add6/1
  [Vq0] -> Add5/2
  Add2/1 -> Add5/1
  Product/1 -> [Vd0]
  Product1/1 -> [Vq0]
  Constant2/1 -> Add4/2
  Add4/1 -> Product1/2
  Gain5/1 -> Add4/1
  [Wm] -> Product/2
  Id/1 -> Subtract/2, Gain5/1
  Gain4/1 -> Product/1
  Switch1/1 -> Gain3/1
  Abs1/1 -> Compare To Constant1/1
  Compare To Constant1/1 -> Switch1/2
  Constant1/1 -> Switch1/3
  Constant/1 -> Switch/3
  Compare To Constant/1 -> Switch/2
  Switch/1 -> Gain1/1
  Add5/1 -> Saturation3/1
  IntregralResetFlag/1 -> Delay One Step1/2, Delay One Step/2
  IqRef/1 -> Subtract1/1
  Iq/1 -> Gain4/1, Subtract1/2
  Gain2/1 -> Add2/1  "IqKp"
  Gain3/1 -> Add3/1
  Delay One Step1/1 -> Add3/2
  Add3/1 -> Saturation1/1  "IqKi"
  Saturation1/1 -> Add2/2, Delay One Step1/1  "IqKiLimit"
  Saturation/1 -> Delay One Step/1, Add/2  "IdKiLimit"
  Add1/1 -> Saturation/1  "IdKi"
  Delay One Step/1 -> Add1/2
  Gain1/1 -> Add1/1
  Abs/1 -> Compare To Constant/1
  Gain/1 -> Add/1  "IdKp"
  Subtract/1 -> currentRController_D/1(CurrErr), Abs/1, Switch/1, Gain/1
  IdRef/1 -> Subtract/1
  currentRController_D/1(UR_Ref) -> Add/3  "UdR_Ref"
  currentRController_Q/1(UR_Ref) -> Add2/3  "UqR_Ref"
  [Wm] -> currentRController_Q/2(Wm)
  Constant3/1 -> currentRController_Q/3(UReal)
  Constant4/1 -> currentRController_D/3(UReal)
  [Wm] -> currentRController_D/2(Wm)

== system MotorCtrl_FOC_Math/HFTask/fluxobservor ==
  Valpha : Inport
  Vbeta : Inport  Port=2
  Ialpha : Inport  Port=3
  Ibeta : Inport  Port=4
  getFlux : Subsystem
  getSpeedandTheta : Subsystem
  Speed : Outport
  Theta : Outport  Port=2
  wires:
  getSpeedandTheta/2(Theta) -> Theta/1
  getSpeedandTheta/1(Speed) -> Speed/1
  getFlux/2(Phibeta) -> getSpeedandTheta/2(Phibeta)
  getFlux/1(Phialpha) -> getSpeedandTheta/1(Phialpha)
  Ibeta/1 -> getFlux/4(Ibeta)
  Ialpha/1 -> getFlux/3(Ialpha)
  Vbeta/1 -> getFlux/2(Vbeta)
  Valpha/1 -> getFlux/1(Valpha)
